simulink model "system3"  (R2023b)
settings: Solver=VariableStepAuto  StartTime=0.0  StopTime=10.0  RelTol=1e-3
undefined symbols (not defined in the file): a, x0
settings Model: Creator=roman  LastModifiedBy=roman

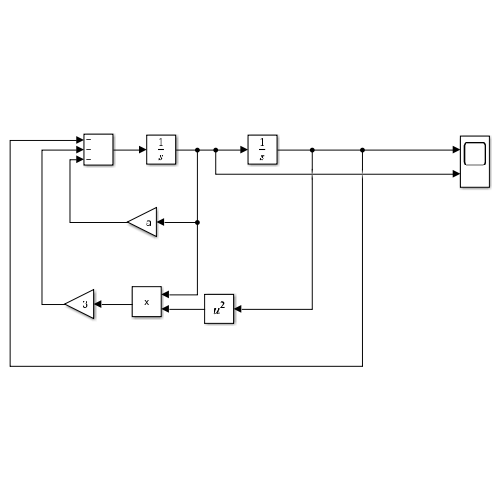
[thumbnail: Simulink's stored preview of the top-level diagram]
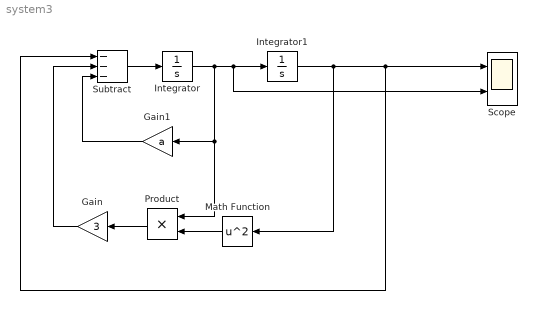
== system system3 ==
  Gain : Gain  Gain=3
  Gain1 : Gain  Gain=a
  Integrator : Integrator  InitialCondition=x0(2)
  Integrator1 : Integrator  InitialCondition=x0(1)
  Math Function : Math  Operator=square
  Product : Product
  Scope : Scope  NumInputPorts=2
  Subtract : Sum  Inputs=---
  wires:
  Integrator/1 -> Gain1/1, Product/1, Scope/2, Integrator1/1
  Integrator1/1 -> Math Function/1, Subtract/1, Scope/1
  Subtract/1 -> Integrator/1
  Math Function/1 -> Product/2
  Product/1 -> Gain/1
  Gain/1 -> Subtract/2
  Gain1/1 -> Subtract/3
